simulink model "TST_AirCtl_CtlValCalc"  (R2016b)
settings: Solver=FixedStepDiscrete  StartTime=0.0  StopTime=simTime  FixedStep=sampleTime  RelTol=1e-3
values from neighbouring files (symbols this model uses):
  testCase = 1    [initTST_AirCtl_CtlValCalc_001.m]
libraries: simulink x3, UnitTest_Lib x1
settings Model: Creator=zhulinfeng  LastModifiedBy=zhulinfeng
settings DebuggingCC: SignalRangeChecking=error

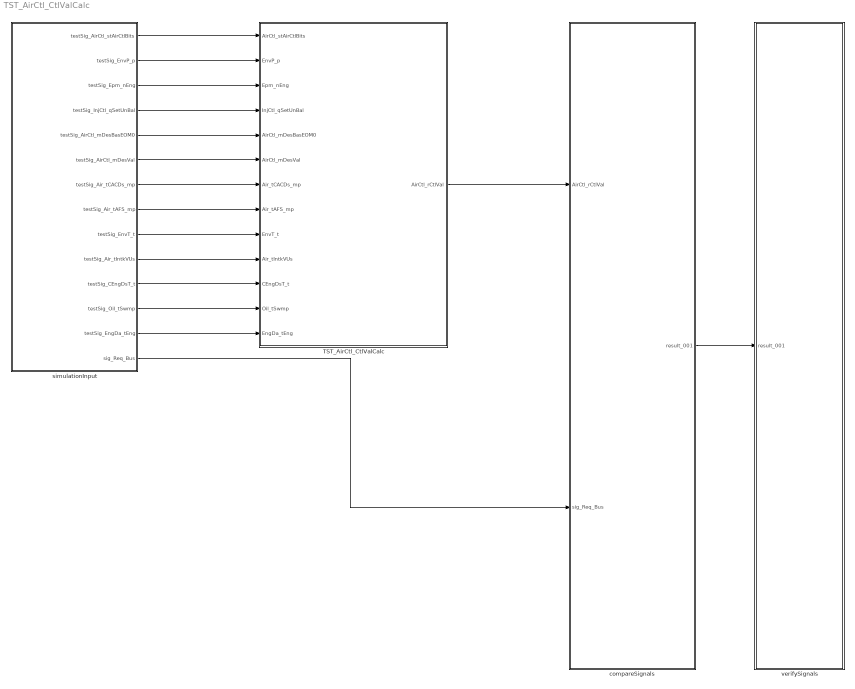
== system TST_AirCtl_CtlValCalc ==
  TST_AirCtl_CtlValCalc : Subsystem
  compareSignals : Subsystem
  simulationInput : Subsystem
  verifySignals : Subsystem
  wires:
  simulationInput/1(testSig_AirCtl_stAirCtlBits) -> TST_AirCtl_CtlValCalc/1(AirCtl_stAirCtlBits)
  simulationInput/2(testSig_EnvP_p) -> TST_AirCtl_CtlValCalc/2(EnvP_p)
  simulationInput/3(testSig_Epm_nEng) -> TST_AirCtl_CtlValCalc/3(Epm_nEng)
  simulationInput/4(testSig_InjCtl_qSetUnBal) -> TST_AirCtl_CtlValCalc/4(InjCtl_qSetUnBal)
  simulationInput/5(testSig_AirCtl_mDesBasEOM0) -> TST_AirCtl_CtlValCalc/5(AirCtl_mDesBasEOM0)
  simulationInput/6(testSig_AirCtl_mDesVal) -> TST_AirCtl_CtlValCalc/6(AirCtl_mDesVal)
  simulationInput/7(testSig_Air_tCACDs_mp) -> TST_AirCtl_CtlValCalc/7(Air_tCACDs_mp)
  simulationInput/8(testSig_Air_tAFS_mp) -> TST_AirCtl_CtlValCalc/8(Air_tAFS_mp)
  simulationInput/9(testSig_EnvT_t) -> TST_AirCtl_CtlValCalc/9(EnvT_t)
  simulationInput/10(testSig_Air_tIntkVUs) -> TST_AirCtl_CtlValCalc/10(Air_tIntkVUs)
  simulationInput/11(testSig_CEngDsT_t) -> TST_AirCtl_CtlValCalc/11(CEngDsT_t)
  simulationInput/12(testSig_Oil_tSwmp) -> TST_AirCtl_CtlValCalc/12(Oil_tSwmp)
  simulationInput/13(testSig_EngDa_tEng) -> TST_AirCtl_CtlValCalc/13(EngDa_tEng)
  TST_AirCtl_CtlValCalc/1(AirCtl_rCtlVal) -> compareSignals/1(AirCtl_rCtlVal)
  simulationInput/14(sig_Req_Bus) -> compareSignals/2(sig_Req_Bus)
  compareSignals/1(result_001) -> verifySignals/1(result_001)

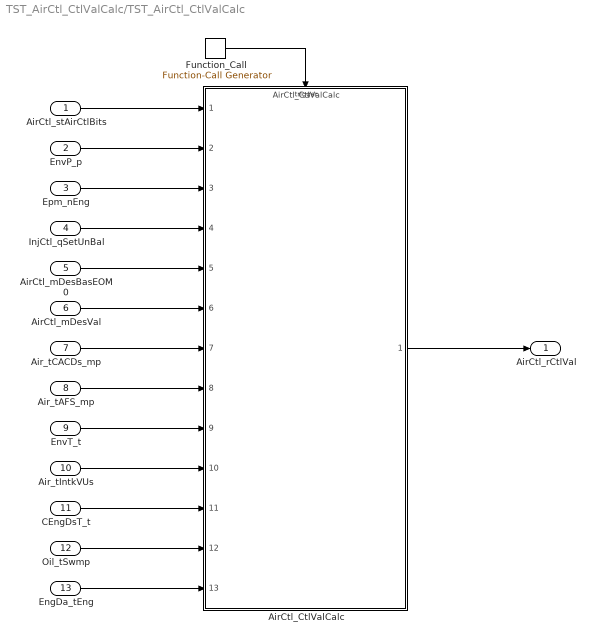
== system TST_AirCtl_CtlValCalc/TST_AirCtl_CtlValCalc ==
  AirCtl_stAirCtlBits : Inport
  EnvP_p : Inport  Port=2
  Epm_nEng : Inport  Port=3
  InjCtl_qSetUnBal : Inport  Port=4
  AirCtl_mDesBasEOM0 : Inport  Port=5
  AirCtl_mDesVal : Inport  Port=6
  Air_tCACDs_mp : Inport  Port=7
  Air_tAFS_mp : Inport  Port=8
  EnvT_t : Inport  Port=9
  Air_tIntkVUs : Inport  Port=10
  CEngDsT_t : Inport  Port=11
  Oil_tSwmp : Inport  Port=12
  EngDa_tEng : Inport  Port=13
  AirCtl_CtlValCalc : ModelReference  ModelNameDialog=AirCtl_CtlValCalc  SimulationMode=Normal  ModelReferenceVersion=1.17  TriggerPortName=function  TriggerPortTriggerType=function-call  TriggerPortStatesWhenEnabling=held
  Function_Call : simulink/Ports & Subsystems/Function-Call Generator  sample_time=sampleTime  numberOfIterations=1
  AirCtl_rCtlVal : Outport
  wires:
  Function_Call/1 -> AirCtl_CtlValCalc/Trigger
  AirCtl_stAirCtlBits/1 -> AirCtl_CtlValCalc/1
  EnvP_p/1 -> AirCtl_CtlValCalc/2
  Epm_nEng/1 -> AirCtl_CtlValCalc/3
  InjCtl_qSetUnBal/1 -> AirCtl_CtlValCalc/4
  AirCtl_mDesBasEOM0/1 -> AirCtl_CtlValCalc/5
  AirCtl_mDesVal/1 -> AirCtl_CtlValCalc/6
  Air_tCACDs_mp/1 -> AirCtl_CtlValCalc/7
  Air_tAFS_mp/1 -> AirCtl_CtlValCalc/8
  EnvT_t/1 -> AirCtl_CtlValCalc/9
  Air_tIntkVUs/1 -> AirCtl_CtlValCalc/10
  CEngDsT_t/1 -> AirCtl_CtlValCalc/11
  Oil_tSwmp/1 -> AirCtl_CtlValCalc/12
  EngDa_tEng/1 -> AirCtl_CtlValCalc/13
  AirCtl_CtlValCalc/1 -> AirCtl_rCtlVal/1

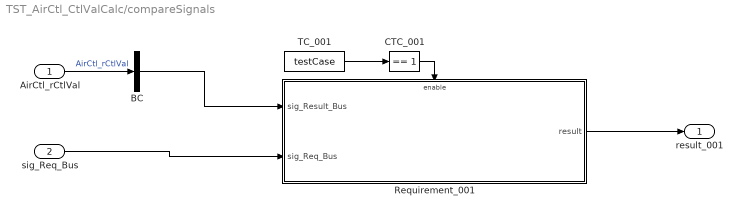
== system TST_AirCtl_CtlValCalc/compareSignals ==
  AirCtl_rCtlVal : Inport
  sig_Req_Bus : Inport  Port=2
  BC : BusCreator  Inputs=1
  CTC_001 : simulink/Logic and Bit Operations/Compare To Constant  relop===  const=1  OutDataTypeStr=boolean
  Requirement_001 : Subsystem
  TC_001 : Constant  Value=testCase
  result_001 : Outport
  wires:
  AirCtl_rCtlVal/1 -> BC/1  "AirCtl_rCtlVal"
  TC_001/1 -> CTC_001/1
  CTC_001/1 -> Requirement_001/Enable
  sig_Req_Bus/1 -> Requirement_001/2(sig_Req_Bus)
  BC/1 -> Requirement_001/1(sig_Result_Bus)
  Requirement_001/1(result) -> result_001/1

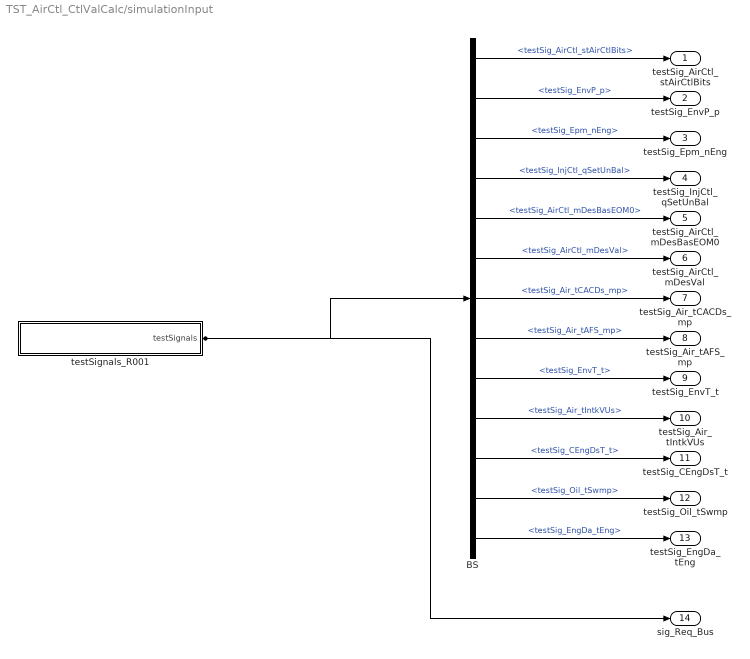
== system TST_AirCtl_CtlValCalc/simulationInput ==
  BS : BusSelector  OutputSignals=testSig_AirCtl_stAirCtlBits,testSig_EnvP_p,testSig_Epm_nEng,testSig_InjCtl_qSetUnBal,testSig_AirCtl_mDesBasEOM0,testSig_AirCtl_mDesVal,testSig_Air_tCACDs_mp,testSig_Air_tAFS_mp,testSig_EnvT_t,testSig_Air_tIntkVUs,testSig_CEngDsT_t,testSig_Oil_tSwmp,testSig_EngDa_tEng
  testSignals_R001 : Subsystem
  testSig_AirCtl_stAirCtlBits : Outport
  testSig_EnvP_p : Outport  Port=2
  testSig_Epm_nEng : Outport  Port=3
  testSig_InjCtl_qSetUnBal : Outport  Port=4
  testSig_AirCtl_mDesBasEOM0 : Outport  Port=5
  testSig_AirCtl_mDesVal : Outport  Port=6
  testSig_Air_tCACDs_mp : Outport  Port=7
  testSig_Air_tAFS_mp : Outport  Port=8
  testSig_EnvT_t : Outport  Port=9
  testSig_Air_tIntkVUs : Outport  Port=10
  testSig_CEngDsT_t : Outport  Port=11
  testSig_Oil_tSwmp : Outport  Port=12
  testSig_EngDa_tEng : Outport  Port=13
  sig_Req_Bus : Outport  Port=14
  wires:
  BS/1 -> testSig_AirCtl_stAirCtlBits/1  "<testSig_AirCtl_stAirCtlBits>"
  BS/2 -> testSig_EnvP_p/1  "<testSig_EnvP_p>"
  BS/3 -> testSig_Epm_nEng/1  "<testSig_Epm_nEng>"
  BS/4 -> testSig_InjCtl_qSetUnBal/1  "<testSig_InjCtl_qSetUnBal>"
  BS/5 -> testSig_AirCtl_mDesBasEOM0/1  "<testSig_AirCtl_mDesBasEOM0>"
  BS/6 -> testSig_AirCtl_mDesVal/1  "<testSig_AirCtl_mDesVal>"
  BS/7 -> testSig_Air_tCACDs_mp/1  "<testSig_Air_tCACDs_mp>"
  BS/8 -> testSig_Air_tAFS_mp/1  "<testSig_Air_tAFS_mp>"
  BS/9 -> testSig_EnvT_t/1  "<testSig_EnvT_t>"
  BS/10 -> testSig_Air_tIntkVUs/1  "<testSig_Air_tIntkVUs>"
  BS/11 -> testSig_CEngDsT_t/1  "<testSig_CEngDsT_t>"
  BS/12 -> testSig_Oil_tSwmp/1  "<testSig_Oil_tSwmp>"
  BS/13 -> testSig_EngDa_tEng/1  "<testSig_EngDa_tEng>"
  testSignals_R001/1(testSignals) -> BS/1, sig_Req_Bus/1

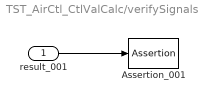
== system TST_AirCtl_CtlValCalc/verifySignals ==
  result_001 : Inport
  Assertion_001 : Assertion  Enabled=off
  wires:
  result_001/1 -> Assertion_001/1

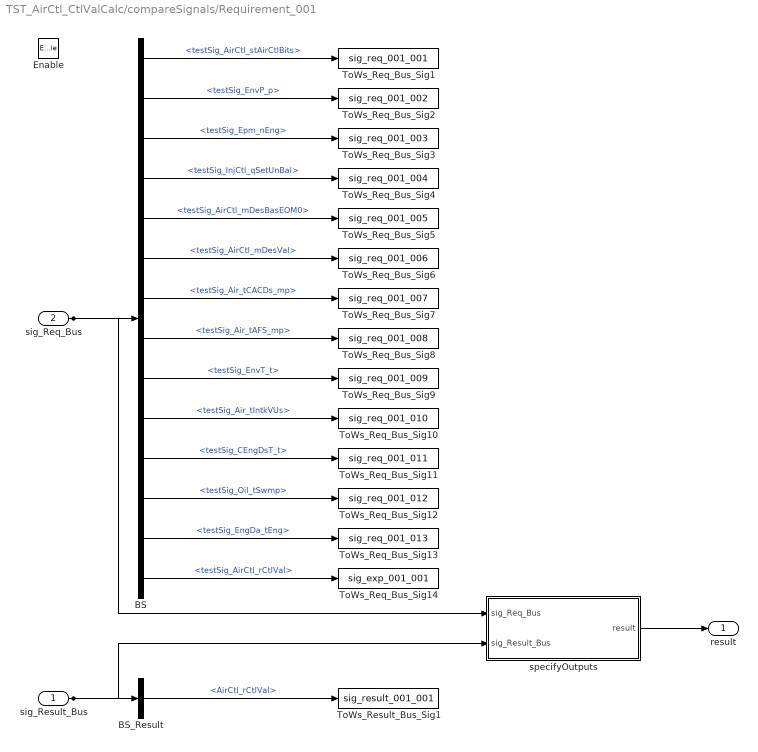
== system TST_AirCtl_CtlValCalc/compareSignals/Requirement_001 ==
  sig_Result_Bus : Inport
  sig_Req_Bus : Inport  Port=2
  Enable : EnablePort
  BS : BusSelector  OutputSignals=testSig_AirCtl_stAirCtlBits,testSig_EnvP_p,testSig_Epm_nEng,testSig_InjCtl_qSetUnBal,testSig_AirCtl_mDesBasEOM0,testSig_AirCtl_mDesVal,testSig_Air_tCACDs_mp,testSig_Air_tAFS_mp,testSig_EnvT_t,testSig_Air_tIntkVUs,testSig_CEngDsT_t,testSig_Oil_tSwmp,testSig_EngDa_tEng,testSig_AirCtl_rCtlVal
  BS_Result : BusSelector  OutputSignals=AirCtl_rCtlVal
  ToWs_Req_Bus_Sig1 : ToWorkspace  VariableName=sig_req_001_001  SaveFormat=Structure With Time
  ToWs_Req_Bus_Sig10 : ToWorkspace  VariableName=sig_req_001_010  SaveFormat=Structure With Time
  ToWs_Req_Bus_Sig11 : ToWorkspace  VariableName=sig_req_001_011  SaveFormat=Structure With Time
  ToWs_Req_Bus_Sig12 : ToWorkspace  VariableName=sig_req_001_012  SaveFormat=Structure With Time
  ToWs_Req_Bus_Sig13 : ToWorkspace  VariableName=sig_req_001_013  SaveFormat=Structure With Time
  ToWs_Req_Bus_Sig14 : ToWorkspace  VariableName=sig_exp_001_001  SaveFormat=Structure With Time
  ToWs_Req_Bus_Sig2 : ToWorkspace  VariableName=sig_req_001_002  SaveFormat=Structure With Time
  ToWs_Req_Bus_Sig3 : ToWorkspace  VariableName=sig_req_001_003  SaveFormat=Structure With Time
  ToWs_Req_Bus_Sig4 : ToWorkspace  VariableName=sig_req_001_004  SaveFormat=Structure With Time
  ToWs_Req_Bus_Sig5 : ToWorkspace  VariableName=sig_req_001_005  SaveFormat=Structure With Time
  ToWs_Req_Bus_Sig6 : ToWorkspace  VariableName=sig_req_001_006  SaveFormat=Structure With Time
  ToWs_Req_Bus_Sig7 : ToWorkspace  VariableName=sig_req_001_007  SaveFormat=Structure With Time
  ToWs_Req_Bus_Sig8 : ToWorkspace  VariableName=sig_req_001_008  SaveFormat=Structure With Time
  ToWs_Req_Bus_Sig9 : ToWorkspace  VariableName=sig_req_001_009  SaveFormat=Structure With Time
  ToWs_Result_Bus_Sig1 : ToWorkspace  VariableName=sig_result_001_001  SaveFormat=Structure With Time
  specifyOutputs : Subsystem
  result : Outport
  wires:
  sig_Req_Bus/1 -> BS/1, specifyOutputs/1(sig_Req_Bus)
  BS/1 -> ToWs_Req_Bus_Sig1/1  "<testSig_AirCtl_stAirCtlBits>"
  BS/2 -> ToWs_Req_Bus_Sig2/1  "<testSig_EnvP_p>"
  BS/3 -> ToWs_Req_Bus_Sig3/1  "<testSig_Epm_nEng>"
  BS/4 -> ToWs_Req_Bus_Sig4/1  "<testSig_InjCtl_qSetUnBal>"
  BS/5 -> ToWs_Req_Bus_Sig5/1  "<testSig_AirCtl_mDesBasEOM0>"
  BS/6 -> ToWs_Req_Bus_Sig6/1  "<testSig_AirCtl_mDesVal>"
  BS/7 -> ToWs_Req_Bus_Sig7/1  "<testSig_Air_tCACDs_mp>"
  BS/8 -> ToWs_Req_Bus_Sig8/1  "<testSig_Air_tAFS_mp>"
  BS/9 -> ToWs_Req_Bus_Sig9/1  "<testSig_EnvT_t>"
  BS/10 -> ToWs_Req_Bus_Sig10/1  "<testSig_Air_tIntkVUs>"
  BS/11 -> ToWs_Req_Bus_Sig11/1  "<testSig_CEngDsT_t>"
  BS/12 -> ToWs_Req_Bus_Sig12/1  "<testSig_Oil_tSwmp>"
  BS/13 -> ToWs_Req_Bus_Sig13/1  "<testSig_EngDa_tEng>"
  BS/14 -> ToWs_Req_Bus_Sig14/1  "<testSig_AirCtl_rCtlVal>"
  sig_Result_Bus/1 -> BS_Result/1, specifyOutputs/2(sig_Result_Bus)
  BS_Result/1 -> ToWs_Result_Bus_Sig1/1  "<AirCtl_rCtlVal>"
  specifyOutputs/1(result) -> result/1

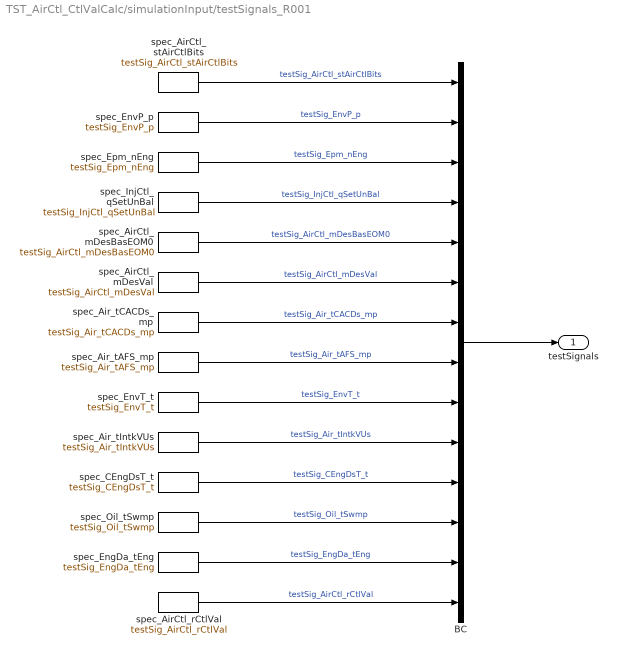
== system TST_AirCtl_CtlValCalc/simulationInput/testSignals_R001 ==
  BC : BusCreator  Inputs=14
  spec_AirCtl_mDesBasEOM0 : FromWorkspace  VariableName=testSig_AirCtl_mDesBasEOM0  Interpolate=off  OutputAfterFinalValue=Holding final value
  spec_AirCtl_mDesVal : FromWorkspace  VariableName=testSig_AirCtl_mDesVal  Interpolate=off  OutputAfterFinalValue=Holding final value
  spec_AirCtl_rCtlVal : FromWorkspace  VariableName=testSig_AirCtl_rCtlVal  Interpolate=off  OutputAfterFinalValue=Holding final value
  spec_AirCtl_stAirCtlBits : FromWorkspace  VariableName=testSig_AirCtl_stAirCtlBits  Interpolate=off  OutputAfterFinalValue=Holding final value
  spec_Air_tAFS_mp : FromWorkspace  VariableName=testSig_Air_tAFS_mp  Interpolate=off  OutputAfterFinalValue=Holding final value
  spec_Air_tCACDs_mp : FromWorkspace  VariableName=testSig_Air_tCACDs_mp  Interpolate=off  OutputAfterFinalValue=Holding final value
  spec_Air_tIntkVUs : FromWorkspace  VariableName=testSig_Air_tIntkVUs  Interpolate=off  OutputAfterFinalValue=Holding final value
  spec_CEngDsT_t : FromWorkspace  VariableName=testSig_CEngDsT_t  Interpolate=off  OutputAfterFinalValue=Holding final value
  spec_EngDa_tEng : FromWorkspace  VariableName=testSig_EngDa_tEng  Interpolate=off  OutputAfterFinalValue=Holding final value
  spec_EnvP_p : FromWorkspace  VariableName=testSig_EnvP_p  Interpolate=off  OutputAfterFinalValue=Holding final value
  spec_EnvT_t : FromWorkspace  VariableName=testSig_EnvT_t  Interpolate=off  OutputAfterFinalValue=Holding final value
  spec_Epm_nEng : FromWorkspace  VariableName=testSig_Epm_nEng  Interpolate=off  OutputAfterFinalValue=Holding final value
  spec_InjCtl_qSetUnBal : FromWorkspace  VariableName=testSig_InjCtl_qSetUnBal  Interpolate=off  OutputAfterFinalValue=Holding final value
  spec_Oil_tSwmp : FromWorkspace  VariableName=testSig_Oil_tSwmp  Interpolate=off  OutputAfterFinalValue=Holding final value
  testSignals : Outport
  wires:
  BC/1 -> testSignals/1
  spec_AirCtl_stAirCtlBits/1 -> BC/1  "testSig_AirCtl_stAirCtlBits"
  spec_EnvP_p/1 -> BC/2  "testSig_EnvP_p"
  spec_Epm_nEng/1 -> BC/3  "testSig_Epm_nEng"
  spec_InjCtl_qSetUnBal/1 -> BC/4  "testSig_InjCtl_qSetUnBal"
  spec_AirCtl_mDesBasEOM0/1 -> BC/5  "testSig_AirCtl_mDesBasEOM0"
  spec_AirCtl_mDesVal/1 -> BC/6  "testSig_AirCtl_mDesVal"
  spec_Air_tCACDs_mp/1 -> BC/7  "testSig_Air_tCACDs_mp"
  spec_Air_tAFS_mp/1 -> BC/8  "testSig_Air_tAFS_mp"
  spec_EnvT_t/1 -> BC/9  "testSig_EnvT_t"
  spec_Air_tIntkVUs/1 -> BC/10  "testSig_Air_tIntkVUs"
  spec_CEngDsT_t/1 -> BC/11  "testSig_CEngDsT_t"
  spec_Oil_tSwmp/1 -> BC/12  "testSig_Oil_tSwmp"
  spec_EngDa_tEng/1 -> BC/13  "testSig_EngDa_tEng"
  spec_AirCtl_rCtlVal/1 -> BC/14  "testSig_AirCtl_rCtlVal"

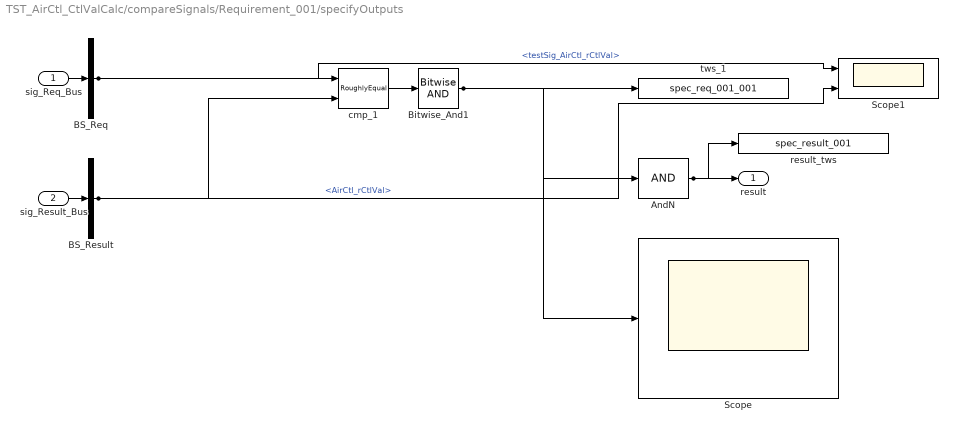
== system TST_AirCtl_CtlValCalc/compareSignals/Requirement_001/specifyOutputs ==
  sig_Req_Bus : Inport
  sig_Result_Bus : Inport  Port=2
  AndN : Logic  Inputs=1
  BS_Req : BusSelector  OutputSignals=testSig_AirCtl_rCtlVal
  BS_Result : BusSelector  OutputSignals=AirCtl_rCtlVal
  Bitwise_And1 : simulink/Logic and Bit Operations/Bitwise Operator  logicop=AND  UseBitMask=off  BitMask=bin2dec('11011001')  BitMaskRealWorld=Stored Integer
  Scope : Scope
  Scope1 : Scope  NumInputPorts=2
  cmp_1 : UnitTest_Lib/RoughlyEqual  slope=0.1
  result_tws : ToWorkspace  VariableName=spec_result_001
  tws_1 : ToWorkspace  VariableName=spec_req_001_001
  result : Outport
  wires:
  sig_Req_Bus/1 -> BS_Req/1
  sig_Result_Bus/1 -> BS_Result/1
  AndN/1 -> result/1, result_tws/1
  BS_Req/1 -> cmp_1/1, Scope1/1  "<testSig_AirCtl_rCtlVal>"
  BS_Result/1 -> cmp_1/2, Scope1/2  "<AirCtl_rCtlVal>"
  cmp_1/1 -> Bitwise_And1/1
  Bitwise_And1/1 -> tws_1/1, AndN/1, Scope/1
